simulink model "TESTES"  (R2017a)
settings: Solver=VariableStepAuto  StartTime=0.0  StopTime=1  RelTol=1e-3
libraries: powerlib_meascontrol x1
settings Model: Creator=gabrielrodrigues  LastModifiedBy=gabrielrodrigues

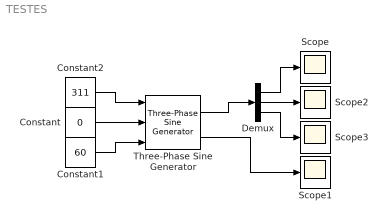
== system TESTES ==
  Constant : Constant  Value=0
  Constant1 : Constant  Value=60
  Constant2 : Constant  Value=311
  Demux : Demux  Outputs=3
  Scope{,1..3} (4 alike) : Scope
  Three-Phase Sine Generator : powerlib_meascontrol/Pulse & Signal Generators/Three-Phase Sine Generator  Ts=1e-6
      settings: SourceProductName=Simscape Power Systems  SourceProductBaseCode=PS
  wires:
  Constant/1 -> Three-Phase Sine Generator/2
  Constant1/1 -> Three-Phase Sine Generator/3
  Constant2/1 -> Three-Phase Sine Generator/1
  Three-Phase Sine Generator/1 -> Demux/1
  Three-Phase Sine Generator/2 -> Scope1/1
  Demux/1 -> Scope/1
  Demux/2 -> Scope2/1
  Demux/3 -> Scope3/1
